simulink model "hw2_2_mdl"  (R2024b)
settings: Solver=ode4  StartTime=0.0  StopTime=simTime  FixedStep=sampling_time  RelTol=1e-3
values from neighbouring files (symbols this model uses):
  A = [0 1 ... (first row only)    [hw2_2.m]
  Am = [0 1 ... (first row only)    [hw2_2.m]
  B = [0; b]    [hw2_2.m]
  Bm = [0; 5]    [hw2_2.m]
  C = [1 0 ... (first row only)    [hw2_2.m]
  Cm = [1 0 ... (first row only)    [hw2_2.m]
  D = [0; 0]    [hw2_2.m]
  Dm = [0; 0]    [hw2_2.m]
  gamma1 = 1    [hw2_1.m]    (also in hw2_2.m)
  gamma2 = 1    [hw2_1.m]    (also in hw2_2.m)
  inputMagnitude = 1    [hw2_1.m]    (also in hw2_2.m)
settings Model: Creator=kemal  LastModifiedBy=kemal

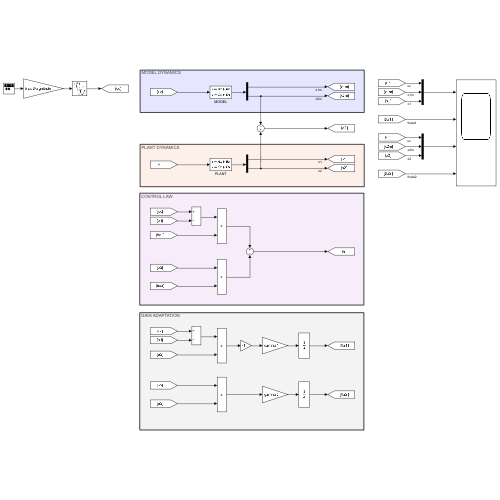
[thumbnail: Simulink's stored preview of the top-level diagram]
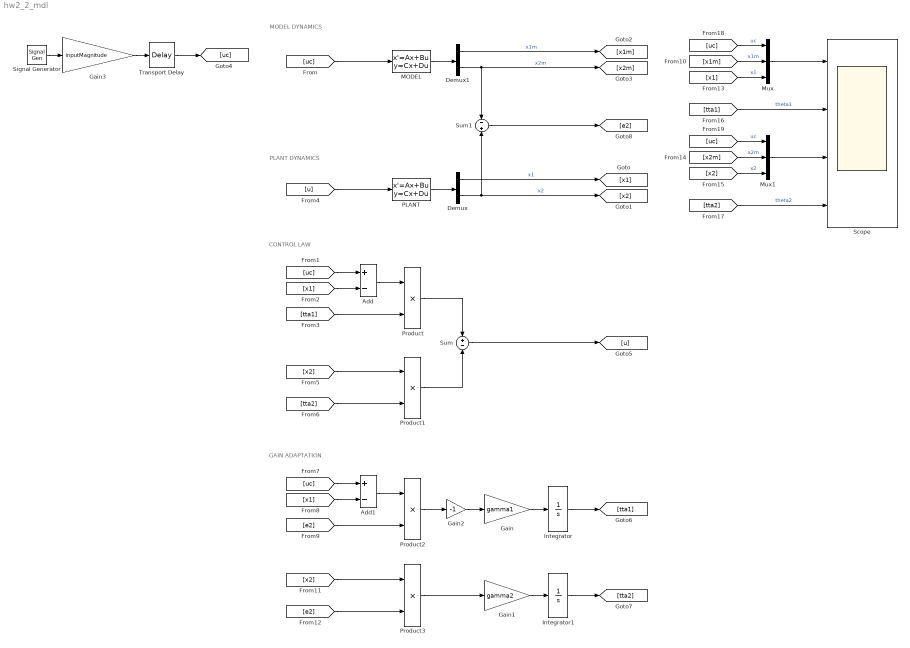
== system hw2_2_mdl ==
  note: GAIN ADAPTATION
  note: CONTROL LAW
  note: MODEL DYNAMICS
  note: PLANT DYNAMICS
  Add : Sum  Inputs=+-
  Add1 : Sum  Inputs=+-
  Demux : Demux  Outputs=2
  Demux1 : Demux  Outputs=2
  Gain : Gain  Gain=gamma1
  Gain1 : Gain  Gain=gamma2
  Gain2 : Gain  Gain=-1
  Gain3 : Gain  Gain=inputMagnitude
  Integrator : Integrator
  Integrator1 : Integrator
  MODEL : StateSpace  A=Am  B=Bm  C=Cm  D=Dm  InitialCondition=0
  Mux : Mux  Inputs=3
  Mux1 : Mux  Inputs=3
  PLANT : StateSpace  A=A  B=B  C=C  D=D  InitialCondition=0
  Product{,1..3} (4 alike) : Product
  Scope : Scope  NumInputPorts=4
  Signal Generator : SignalGenerator  WaveForm=square  Frequency=0.1
  Sum : Sum  Inputs=+-
  Sum1 : Sum  Inputs=-+
  Transport Delay : TransportDelay  DelayTime=5
  wires:
  PLANT/1 -> Demux/1
  MODEL/1 -> Demux1/1
  Demux/1 -> [x1]  "x1"
  Demux/2 -> [x2], Sum1/2  "x2"
  Demux1/2 -> [x2m], Sum1/1  "x2m"
  Demux1/1 -> [x1m]  "x1m"
  [uc] -> MODEL/1
  [uc] -> Add/1
  [x1] -> Add/2
  Add/1 -> Product/1
  [tta1] -> Product/2
  Product/1 -> Sum/1
  [tta2] -> Product1/2
  [x2] -> Product1/1
  Product1/1 -> Sum/2
  Sum/1 -> [u]
  Signal Generator/1 -> Gain3/1
  [u] -> PLANT/1
  Integrator/1 -> [tta1]
  [x1] -> Add1/2
  [uc] -> Add1/1
  Sum1/1 -> [e2]
  Add1/1 -> Product2/1
  [e2] -> Product2/2
  Product2/1 -> Gain2/1
  Gain/1 -> Integrator/1
  Gain1/1 -> Integrator1/1
  Product3/1 -> Gain1/1
  [e2] -> Product3/2
  [x2] -> Product3/1
  Integrator1/1 -> [tta2]
  Gain2/1 -> Gain/1
  [x1m] -> Mux/2  "x1m"
  [x1] -> Mux/3  "x1"
  [x2m] -> Mux1/2  "x2m"
  [x2] -> Mux1/3  "x2"
  Mux/1 -> Scope/1
  [tta1] -> Scope/2  "theta1"
  [tta2] -> Scope/4  "theta2"
  [uc] -> Mux/1  "uc"
  Transport Delay/1 -> [uc]
  [uc] -> Mux1/1  "uc"
  Mux1/1 -> Scope/3
  Gain3/1 -> Transport Delay/1
